simulink model "lab2_model1"  (R2021b)
settings: Solver=FixedStepAuto  StartTime=0.0  StopTime=60  FixedStep=0.001  RelTol=1e-3
libraries: cstblocks x2, qube2servo x2
settings Model: Creator=12288  LastModifiedBy=12288

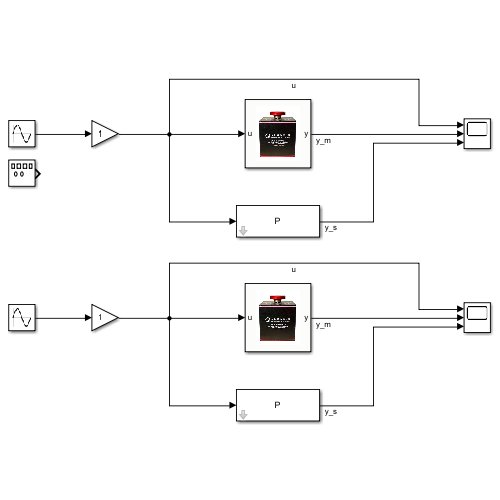
[thumbnail: Simulink's stored preview of the top-level diagram]
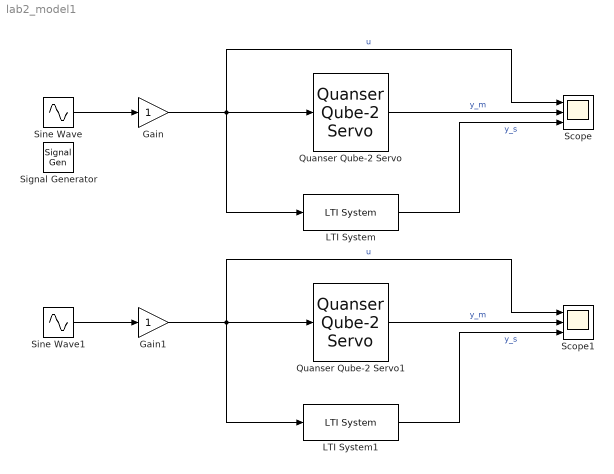
== system lab2_model1 ==
  Gain : Gain
  Gain1 : Gain
  LTI System : cstblocks/LTI System  sys=P  IC=[]
  LTI System1 : cstblocks/LTI System  sys=P  IC=[]
  Quanser Qube-2 Servo : qube2servo/Quanser Qube-2 Servo  SystemSampleTime=-1  VariantActivationTime=update diagram  Latency=0  AutoFrameSizeCalculation=off
  Quanser Qube-2 Servo1 : qube2servo/Quanser Qube-2 Servo  SystemSampleTime=-1  VariantActivationTime=update diagram  Latency=0  AutoFrameSizeCalculation=off
  Scope : Scope  NumInputPorts=3
  Scope1 : Scope  NumInputPorts=3
  Signal Generator : SignalGenerator  Units=rad/sec
  Sine Wave : Sin  Phase=pi/2  SampleTime=0
  Sine Wave1 : Sin  Frequency=5  Phase=pi/2  SampleTime=0
  wires:
  Gain/1 -> Scope/1, LTI System/1, Quanser Qube-2 Servo/1  "u"
  Quanser Qube-2 Servo/1 -> Scope/2  "y_m"
  LTI System/1 -> Scope/3  "y_s"
  Gain1/1 -> Scope1/1, LTI System1/1, Quanser Qube-2 Servo1/1  "u"
  LTI System1/1 -> Scope1/3  "y_s"
  Quanser Qube-2 Servo1/1 -> Scope1/2  "y_m"
  Sine Wave1/1 -> Gain1/1
  Sine Wave/1 -> Gain/1
